simulink model "TDOF_simulink"  (R2026a)
settings: Solver=VariableStepAuto  StopTime=30  MaxStep=1e-3
InitFcn:
  | model_path = fileparts(get_param(bdroot, 'FileName'));
  | parent_path = fileparts(model_path);
  | run(fullfile(parent_path, 'scripts', 'InitFcn.m'));
undefined symbols (not defined in the file): alpha_unique, cd_avg, CG_vec, cn_avg, dI_dt_vec, I_vec, Mach_unique1, S, thrust_vec, time_vec, tot_mass_vec
libraries: aerolibatmos2 x1, aerolibasang x1
settings Model: Creator=awint  LastModifiedBy=benjaminbrobst

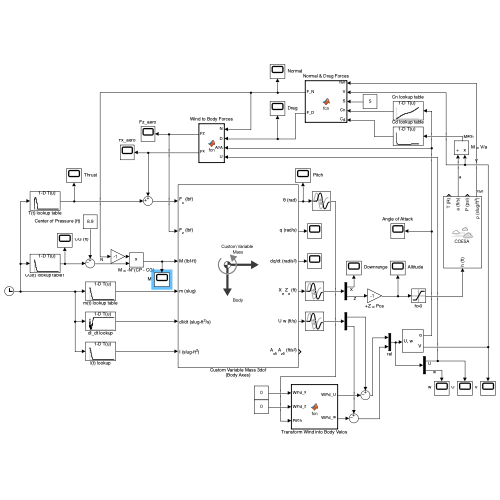
[thumbnail: Simulink's stored preview of the top-level diagram]
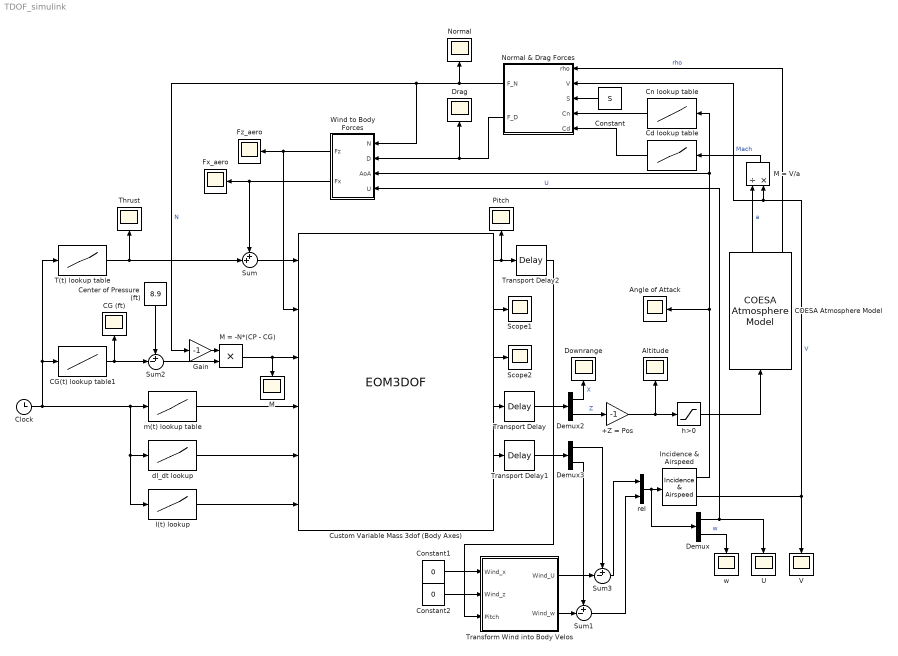
== system TDOF_simulink ==
  +Z = Pos : Gain  Gain=-1
  Altitude : Scope
      settings: ActiveDisplayYMinimum=-635.764520542167  ActiveDisplayYMaximum=5721.8795106507005  DataLoggingVariableName=ScopeData3
  Angle of Attack : Scope
      settings: ActiveDisplayYMinimum=-2.37000408204062  ActiveDisplayYMaximum=3.734571628119034  DataLoggingVariableName=ScopeData18
  CG (ft) : Scope
      settings: ActiveDisplayYMinimum=-1  ActiveDisplayYMaximum=1  DataLoggingVariableName=ScopeData13
  CG(t) lookup table1 : Lookup_n-D  NumberOfTableDimensions=1  BreakpointsForDimension1=time_vec  Table=CG_vec  ExtrapMethod=Clip  UseLastTableValue=on  InternalRulePriority=Speed  RndMeth=Simplest
  COESA Atmosphere Model : aerolibatmos2/COESA Atmosphere Model  units=English (Velocity in ft/s)  spec=1976 COESA-extended U.S. Standard Atmosphere  model=Profile  profile_var=High temperature  profile_percent=1%  profile_alt=5 km (16404 ft)  envelope_var=High temperature  envelope_percent=1%  action=Warning
  Cd lookup table : Lookup_n-D  NumberOfTableDimensions=1  BreakpointsForDimension1=Mach_unique1  Table=cd_avg  ExtrapMethod=Clip  InternalRulePriority=Speed  RndMeth=Simplest
  Center of Pressure (ft) : Constant  Value=8.9
  Clock : Clock
  Cn lookup table : Lookup_n-D  NumberOfTableDimensions=1  BreakpointsForDimension1=alpha_unique  Table=cn_avg  ExtrapMethod=Clip  UseLastTableValue=on  InternalRulePriority=Speed  RndMeth=Simplest
  Constant : Constant  Value=S
  Constant1 : Constant  Value=0
  Constant2 : Constant  Value=0
  Custom Variable Mass 3dof (Body Axes) : EOM3DOF  units=English (velocity in ft/s)  mtype=Custom Variable  v_ini=0  theta_ini=deg2rad(90)  g=32.174
  Demux : Demux  Outputs=2
  Demux2 : Demux  Outputs=2
  Demux3 : Demux  Outputs=2
  Downrange : Scope
      settings: ActiveDisplayYMinimum=-19.712497752344422  ActiveDisplayYMaximum=177.18975439039869  DataLoggingVariableName=ScopeData2
  Drag : Scope
      settings: ActiveDisplayYMinimum=-7.5908313434596018  ActiveDisplayYMaximum=68.317482091136426  DataLoggingVariableName=ScopeData6
  Fx_aero : Scope
      settings: ActiveDisplayYMinimum=-124.52423861742473  ActiveDisplayYMaximum=123.81059420565069  DataLoggingVariableName=ScopeData11
  Fz_aero : Scope
      settings: ActiveDisplayYMinimum=-109.44990928252216  ActiveDisplayYMaximum=112.0429427750761  DataLoggingVariableName=ScopeData12
  Gain : Gain  Gain=-1
  I(t) lookup : Lookup_n-D  NumberOfTableDimensions=1  BreakpointsForDimension1=time_vec  Table=I_vec  ExtrapMethod=Clip  UseLastTableValue=on  InternalRulePriority=Speed  RndMeth=Simplest
  Incidence & Airspeed : aerolibasang/Incidence  & Airspeed
  M : Scope
      settings: ActiveDisplayYMinimum=-217.34060747370111  ActiveDisplayYMaximum=213.49591684829502  DataLoggingVariableName=ScopeData15
  M = -N*(CP - CG) : Product
  M = V/a : Product  Inputs=/*
  Normal : Scope
      settings: ActiveDisplayYMinimum=-25.126869567561766  ActiveDisplayYMaximum=23.773786342021697  DataLoggingVariableName=ScopeData5
  Normal & Drag Forces : MATLAB Function  TreatAsAtomicUnit=on
  Pitch : Scope
      settings: ActiveDisplayYMinimum=-3.926629287237243  ActiveDisplayYMaximum=3.9265258826990146  DataLoggingVariableName=ScopeData8
  Scope1 : Scope
      settings: ActiveDisplayYMinimum=-1  ActiveDisplayYMaximum=1  DataLoggingVariableName=ScopeData16
  Scope2 : Scope
      settings: ActiveDisplayYMinimum=-1  ActiveDisplayYMaximum=1  DataLoggingVariableName=ScopeData17
  Sum : Sum  Inputs=++|
  Sum1 : Sum  Inputs=+-|
  Sum2 : Sum  Inputs=+-|
  Sum3 : Sum  Inputs=+-|
  T(t) lookup table : Lookup_n-D  NumberOfTableDimensions=1  BreakpointsForDimension1=time_vec  Table=thrust_vec  ExtrapMethod=Clip  UseLastTableValue=on  InternalRulePriority=Speed  RndMeth=Simplest
  Thrust : Scope
      settings: ActiveDisplayYMinimum=-1  ActiveDisplayYMaximum=1  DataLoggingVariableName=ScopeData4
  Transform Wind into Body Velos : MATLAB Function  TreatAsAtomicUnit=on
  Transport Delay : TransportDelay  DelayTime=1e-4
  Transport Delay1 : TransportDelay  DelayTime=1e-4
  Transport Delay2 : TransportDelay  DelayTime=1e-4
  U : Scope
      settings: ActiveDisplayYMinimum=-99.6902781300947  ActiveDisplayYMaximum=743.954846014864  DataLoggingVariableName=ScopeData9
  V : Scope
      settings: ActiveDisplayYMinimum=-3.5718401550394403  ActiveDisplayYMaximum=19.517882789166382
  Wind to Body Forces : MATLAB Function  TreatAsAtomicUnit=on
  dI_dt lookup : Lookup_n-D  NumberOfTableDimensions=1  BreakpointsForDimension1=time_vec(1:end-1)  Table=dI_dt_vec  ExtrapMethod=Clip  UseLastTableValue=on  InternalRulePriority=Speed  RndMeth=Simplest
  h>0 : Saturate  UpperLimit=inf  LowerLimit=0
  m(t) lookup table : Lookup_n-D  NumberOfTableDimensions=1  BreakpointsForDimension1=time_vec  Table=tot_mass_vec  ExtrapMethod=Clip  UseLastTableValue=on  InternalRulePriority=Speed  RndMeth=Simplest
  rel : Mux  Inputs=2
  w : Scope
      settings: ActiveDisplayYMinimum=-262.4859690923642  ActiveDisplayYMaximum=268.97679891729467  DataLoggingVariableName=ScopeData10
  wires:
  Clock/1 -> dI_dt lookup/1, I(t) lookup/1, m(t) lookup table/1, T(t) lookup table/1, CG(t) lookup table1/1
  dI_dt lookup/1 -> Custom Variable Mass 3dof (Body Axes)/5
  I(t) lookup/1 -> Custom Variable Mass 3dof (Body Axes)/6
  Demux2/1 -> Downrange/1  "X"
  Demux2/2 -> +Z = Pos/1  "Z"
  Demux/2 -> w/1  "w"
  m(t) lookup table/1 -> Custom Variable Mass 3dof (Body Axes)/4
  T(t) lookup table/1 -> Sum/2, Thrust/1
  Incidence & Airspeed/2 -> V/1, Normal & Drag Forces/2(V), M = V/a/2  "V"
  M = V/a/1 -> Cd lookup table/1  "Mach"
  Cd lookup table/1 -> Normal & Drag Forces/5(Cd)
  Cn lookup table/1 -> Normal & Drag Forces/4(Cn)
  Normal & Drag Forces/1(F_N) -> Normal/1, Wind to Body Forces/1(N), Gain/1  "N"
  COESA Atmosphere Model/2 -> M = V/a/1  "a"
  Custom Variable Mass 3dof (Body Axes)/1 -> Transport Delay2/1, Pitch/1
  Incidence & Airspeed/1 -> Cn lookup table/1, Wind to Body Forces/3(AoA), Angle of Attack/1
  Sum/1 -> Custom Variable Mass 3dof (Body Axes)/1
  Wind to Body Forces/1(Fz) -> Fz_aero/1, Custom Variable Mass 3dof (Body Axes)/2
  Wind to Body Forces/2(Fx) -> Fx_aero/1, Sum/1
  Custom Variable Mass 3dof (Body Axes)/4 -> Transport Delay/1
  Custom Variable Mass 3dof (Body Axes)/5 -> Transport Delay1/1
  Transport Delay/1 -> Demux2/1
  +Z = Pos/1 -> h>0/1, Altitude/1
  h>0/1 -> COESA Atmosphere Model/1
  Sum2/1 -> M = -N*(CP - CG)/2
  M = -N*(CP - CG)/1 -> Custom Variable Mass 3dof (Body Axes)/3, M/1
  Gain/1 -> M = -N*(CP - CG)/1
  CG(t) lookup table1/1 -> Sum2/2, CG (ft)/1
  Custom Variable Mass 3dof (Body Axes)/2 -> Scope1/1
  Custom Variable Mass 3dof (Body Axes)/3 -> Scope2/1
  Constant1/1 -> Transform Wind into Body Velos/1(Wind_x)
  Transport Delay2/1 -> Transform Wind into Body Velos/3(Pitch)
  Transport Delay1/1 -> Demux3/1
  Demux3/2 -> Sum1/1
  Demux3/1 -> Sum3/1
  Transform Wind into Body Velos/2(Wind_w) -> Sum1/2
  Transform Wind into Body Velos/1(Wind_U) -> Sum3/2
  Constant2/1 -> Transform Wind into Body Velos/2(Wind_z)
  Sum1/1 -> rel/2
  Sum3/1 -> rel/1
  rel/1 -> Demux/1, Incidence & Airspeed/1
  Center of Pressure (ft)/1 -> Sum2/1
  Demux/1 -> Wind to Body Forces/4(U), U/1  "U"
  Constant/1 -> Normal & Drag Forces/3(S)
  COESA Atmosphere Model/4 -> Normal & Drag Forces/1(rho)  "rho"
  Normal & Drag Forces/2(F_D) -> Drag/1, Wind to Body Forces/2(D)

== matlab function TDOF_simulink/Normal & Drag Forces ==
  data: rho input; F_N output; V input; S input; Cn input; Cd input; F_D output
function [F_N, F_D] = fcn(rho, V, S, Cn, Cd)

F_N = 0.5 * rho * V.^2 * S * Cn;
F_D = 0.5 * rho * V.^2 * S * Cd;

== matlab function TDOF_simulink/Wind to Body Forces ==
  data: Fz output; N input; D input; Fx output; AoA input; U input
function [Fz, Fx]= fcn(N, D, AoA, U)
Fx = -D*cos(AoA) + N*sin(AoA);
Fx = -abs(Fx) * (1 - 2*(U < 0)); % Correct sign so drag never creates positive feedback loop
Fz = -D*sin(AoA) - N*cos(AoA);

== matlab function TDOF_simulink/Transform Wind into Body Velos ==
  data: Wind_x input; Wind_z input; Pitch input; Wind_U output; Wind_w output
function [Wind_U, Wind_w] = fcn(Wind_x, Wind_z, Pitch)

Wind_U = Wind_x * cos(Pitch) + Wind_z * sin(Pitch);
Wind_w = -Wind_x * sin(Pitch) + Wind_z * cos(Pitch);
